simulink model "flightController"  (R2015a)
settings: Solver=ode45  StartTime=0.0  StopTime=10.0  RelTol=1e-3
InitFcn:
  | initSimulation
values from neighbouring files (symbols this model uses):
  maxPitch = 20    [initSimulation.m]
undefined symbols (not defined in the file or in its folder): drawAircraft, forces_moments, P, plotmavstatevariables
libraries: simulink_extras x2
settings Model: Creator=Ludger Heide  LastModifiedBy=Ludger Heide

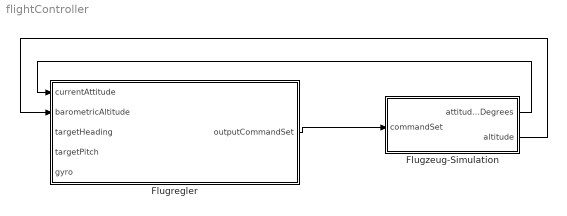
== system flightController ==
  Flugregler : Subsystem  TreatAsAtomicUnit=on
  Flugzeug-Simulation : Subsystem
  wires:
  Flugregler/1(outputCommandSet) -> Flugzeug-Simulation/1(commandSet)
  Flugzeug-Simulation/1(attitudeDegrees) -> Flugregler/1(currentAttitude)
  Flugzeug-Simulation/2(altitude) -> Flugregler/2(barometricAltitude)

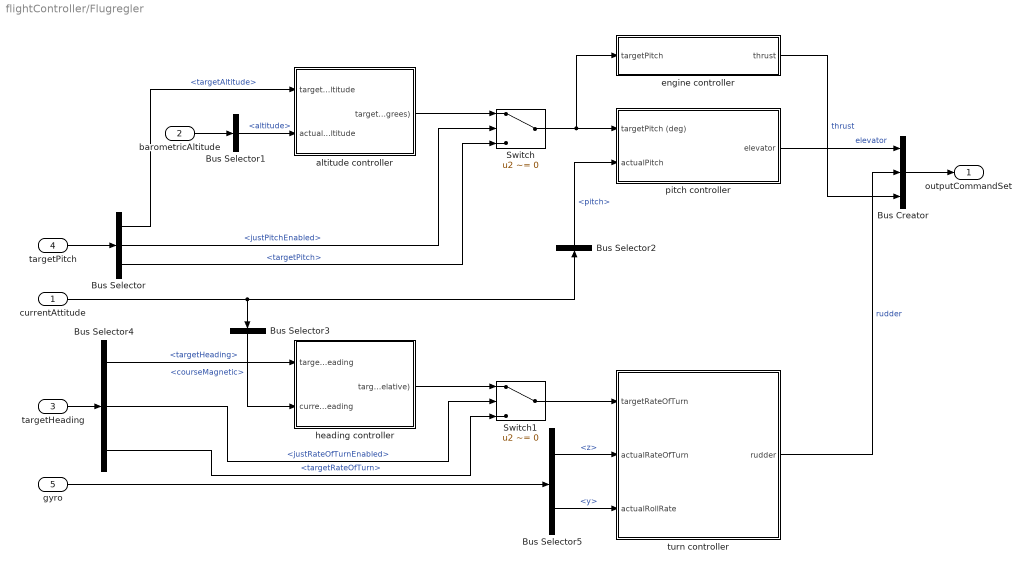
== system flightController/Flugregler ==
  currentAttitude : Inport  OutDataTypeStr=Bus: currentAttitude
  barometricAltitude : Inport  Port=2  OutDataTypeStr=Bus: barometricAltitude
  targetHeading : Inport  Port=3  OutDataTypeStr=Bus: targetHeading
  targetPitch : Inport  Port=4  OutDataTypeStr=Bus: targetPitch
  gyro : Inport  Port=5  OutDataTypeStr=Bus: currentGyro
  Bus Creator : BusCreator  Inputs='elevator','rudder','thrust'  OutDataTypeStr=Bus: outputCommandSet
  Bus Selector : BusSelector  OutputSignals=targetAltitude,justPitchEnabled,targetPitch
  Bus Selector1 : BusSelector  OutputSignals=altitude
  Bus Selector2 : BusSelector  OutputSignals=pitch
  Bus Selector3 : BusSelector  OutputSignals=courseMagnetic
  Bus Selector4 : BusSelector  OutputSignals=targetHeading,justRateOfTurnEnabled,targetRateOfTurn
  Bus Selector5 : BusSelector  OutputSignals=z,y
  Switch : Switch  Criteria=u2 ~= 0
  Switch1 : Switch  Criteria=u2 ~= 0
  altitude controller : Subsystem
  engine controller : Subsystem
  heading controller : Subsystem
  pitch controller : Subsystem
  turn controller : Subsystem
  outputCommandSet : Outport  OutDataTypeStr=Bus: outputCommandSet
  wires:
  Switch/1 -> engine controller/1(targetPitch), pitch controller/1(targetPitch (deg))
  altitude controller/1(targetPitch (degrees)) -> Switch/1
  targetPitch/1 -> Bus Selector/1
  Bus Selector/2 -> Switch/2  "<justPitchEnabled>"
  Bus Selector/3 -> Switch/3  "<targetPitch>"
  Bus Selector/1 -> altitude controller/1(targetAltitude)  "<targetAltitude>"
  barometricAltitude/1 -> Bus Selector1/1
  Bus Selector1/1 -> altitude controller/2(actualAltitude)  "<altitude>"
  Bus Selector2/1 -> pitch controller/2(actualPitch)  "<pitch>"
  currentAttitude/1 -> Bus Selector3/1, Bus Selector2/1
  engine controller/1(thrust) -> Bus Creator/3  "thrust"
  pitch controller/1(elevator) -> Bus Creator/1  "elevator"
  Bus Selector3/1 -> heading controller/2(currentHeading)  "<courseMagnetic>"
  targetHeading/1 -> Bus Selector4/1
  Bus Selector4/1 -> heading controller/1(targetHeading)  "<targetHeading>"
  heading controller/1(targetRateOfTurn (relative)) -> Switch1/1
  Switch1/1 -> turn controller/1(targetRateOfTurn)
  Bus Selector4/2 -> Switch1/2  "<justRateOfTurnEnabled>"
  Bus Selector4/3 -> Switch1/3  "<targetRateOfTurn>"
  turn controller/1(rudder) -> Bus Creator/2  "rudder"
  Bus Creator/1 -> outputCommandSet/1
  Bus Selector5/1 -> turn controller/2(actualRateOfTurn)  "<z>"
  Bus Selector5/2 -> turn controller/3(actualRollRate)  "<y>"
  gyro/1 -> Bus Selector5/1

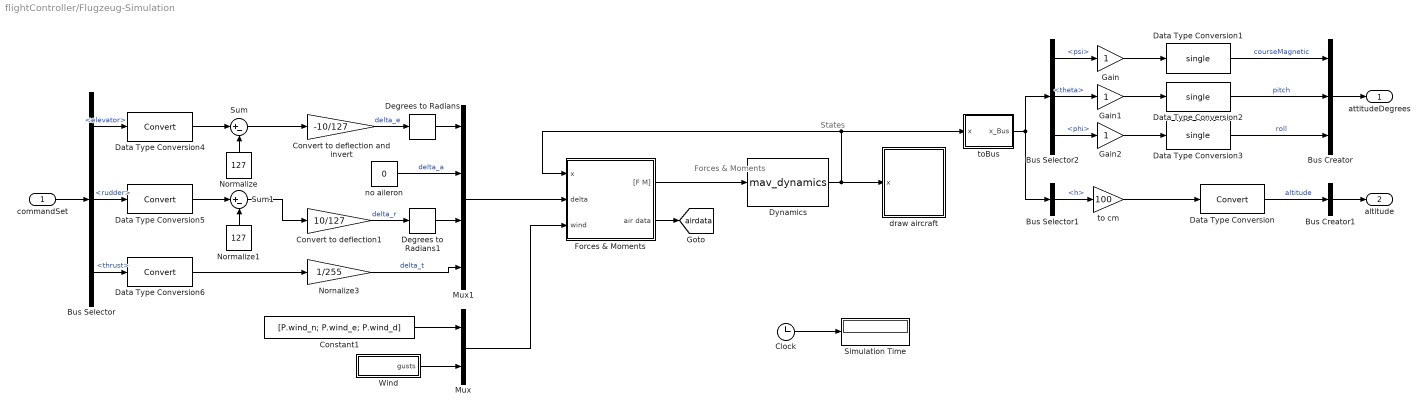
== system flightController/Flugzeug-Simulation ==
  note: Forces & Moments
  note: States
  commandSet : Inport  OutDataTypeStr=Bus: outputCommandSet
  Bus Creator : BusCreator  Inputs='courseMagnetic','pitch','roll'  OutDataTypeStr=Bus: currentAttitude
  Bus Creator1 : BusCreator  Inputs='altitude'  OutDataTypeStr=Bus: barometricAltitude
  Bus Selector : BusSelector  OutputSignals=elevator,rudder,thrust
  Bus Selector1 : BusSelector  OutputSignals=h
  Bus Selector2 : BusSelector  OutputSignals=psi,theta,phi
  Clock : Clock
  Constant1 : Constant  Value=[P.wind_n; P.wind_e; P.wind_d]
  Convert to deflection and invert : Gain  Gain=-10/127
  Convert to deflection1 : Gain  Gain=10/127
  Data Type Conversion{,4..6} (4 alike) : DataTypeConversion
  Data Type Conversion1 : DataTypeConversion  OutDataTypeStr=single
  Data Type Conversion2 : DataTypeConversion  OutDataTypeStr=single
  Data Type Conversion3 : DataTypeConversion  OutDataTypeStr=single
  Degrees to Radians : simulink_extras/Transformations/Degrees to Radians
  Degrees to Radians1 : simulink_extras/Transformations/Degrees to Radians
  Dynamics : S-Function  FunctionName=mav_dynamics  Parameters=P
  Forces & Moments : Subsystem
  Gain : Gain
  Gain1 : Gain
  Gain2 : Gain
  Mux : Mux  Inputs=2
  Mux1 : Mux
  Normalize : Constant  Value=127
  Normalize1 : Constant  Value=127
  Nornalize3 : Gain  Gain=1/255
  Simulation Time : Display
  Sum : Sum  Inputs=|+-
  Sum1 : Sum  Inputs=|+-
  Wind : Subsystem
  draw aircraft : Subsystem
      mask Display: image(imread('tv.jpg'))
  no aileron : Constant  Value=0
  to cm : Gain  Gain=100
  toBus : Subsystem
  attitudeDegrees : Outport  OutDataTypeStr=Bus: currentAttitude
  altitude : Outport  Port=2  OutDataTypeStr=Bus: barometricAltitude
  tag scope: airdata=global
  wires:
  Dynamics/1 -> draw aircraft/1(x), toBus/1(x), Forces & Moments/1(x)
  Convert to deflection1/1 -> Degrees to Radians1/1  "delta_r"
  Convert to deflection and invert/1 -> Degrees to Radians/1  "delta_e"
  Mux1/1 -> Forces & Moments/2(delta)
  Forces & Moments/1("[F M]") -> Dynamics/1
  Clock/1 -> Simulation Time/1
  Mux/1 -> Forces & Moments/3(wind)
  Wind/1(gusts) -> Mux/2
  Constant1/1 -> Mux/1
  Forces & Moments/2(air data) -> [airdata]
  Degrees to Radians/1 -> Mux1/1
  no aileron/1 -> Mux1/2  "delta_a"
  Degrees to Radians1/1 -> Mux1/3
  commandSet/1 -> Bus Selector/1
  Nornalize3/1 -> Mux1/4  "delta_t"
  Bus Selector/1 -> Data Type Conversion4/1  "<elevator>"
  Sum/1 -> Convert to deflection and invert/1
  Normalize/1 -> Sum/2
  Bus Selector/2 -> Data Type Conversion5/1  "<rudder>"
  Sum1/1 -> Convert to deflection1/1
  Normalize1/1 -> Sum1/2
  Bus Selector/3 -> Data Type Conversion6/1  "<thrust>"
  toBus/1(x_Bus) -> Bus Selector2/1, Bus Selector1/1
  Bus Selector2/2 -> Gain1/1  "<theta>"
  Bus Selector2/1 -> Gain/1  "<psi>"
  Bus Selector2/3 -> Gain2/1  "<phi>"
  Gain1/1 -> Data Type Conversion2/1
  Gain2/1 -> Data Type Conversion3/1
  Gain/1 -> Data Type Conversion1/1
  Bus Creator/1 -> attitudeDegrees/1
  to cm/1 -> Data Type Conversion/1
  Bus Selector1/1 -> to cm/1  "<h>"
  Data Type Conversion/1 -> Bus Creator1/1  "altitude"
  Bus Creator1/1 -> altitude/1
  Data Type Conversion1/1 -> Bus Creator/1  "courseMagnetic"
  Data Type Conversion2/1 -> Bus Creator/2  "pitch"
  Data Type Conversion3/1 -> Bus Creator/3  "roll"
  Data Type Conversion4/1 -> Sum/1
  Data Type Conversion5/1 -> Sum1/1
  Data Type Conversion6/1 -> Nornalize3/1

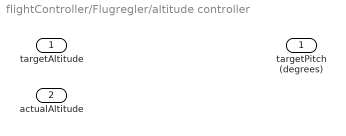
== system flightController/Flugregler/altitude controller ==
  targetAltitude : Inport  OutDataTypeStr=int32
  actualAltitude : Inport  Port=2  OutDataTypeStr=int32
  targetPitch (degrees) : Outport  OutDataTypeStr=int8

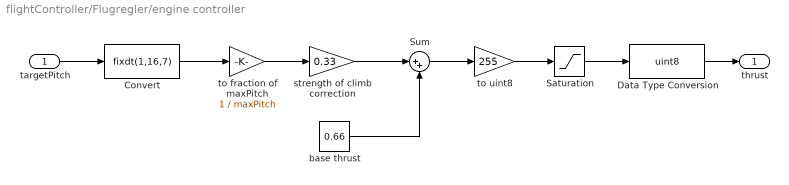
== system flightController/Flugregler/engine controller ==
  targetPitch : Inport  OutDataTypeStr=int8
  Convert : DataTypeConversion  OutMin=-127  OutMax=255  OutDataTypeStr=fixdt(1,16,7)
  Data Type Conversion : DataTypeConversion  OutDataTypeStr=uint8
  Saturation : Saturate  UpperLimit=255  LowerLimit=0
  Sum : Sum  Inputs=|++
  base thrust : Constant  Value=0.66
  strength of climb correction : Gain  Gain=0.33
  to fraction of maxPitch : Gain  Gain=1 / maxPitch
  to uint8 : Gain  Gain=255
  thrust : Outport  OutDataTypeStr=uint8
  wires:
  targetPitch/1 -> Convert/1
  Convert/1 -> to fraction of maxPitch/1
  to fraction of maxPitch/1 -> strength of climb correction/1
  base thrust/1 -> Sum/2
  strength of climb correction/1 -> Sum/1
  Sum/1 -> to uint8/1
  to uint8/1 -> Saturation/1
  Saturation/1 -> Data Type Conversion/1
  Data Type Conversion/1 -> thrust/1

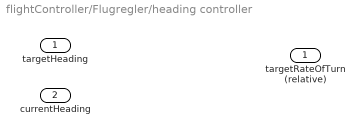
== system flightController/Flugregler/heading controller ==
  targetHeading : Inport  OutDataTypeStr=uint16
  currentHeading : Inport  Port=2  OutDataTypeStr=single
  targetRateOfTurn (relative) : Outport  OutDataTypeStr=int8

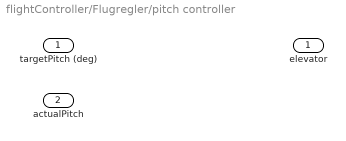
== system flightController/Flugregler/pitch controller ==
  targetPitch (deg) : Inport  OutDataTypeStr=int8
  actualPitch : Inport  Port=2  OutDataTypeStr=single
  elevator : Outport  OutDataTypeStr=uint8

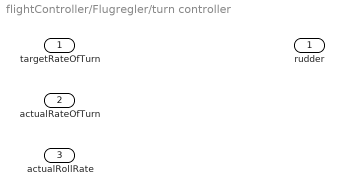
== system flightController/Flugregler/turn controller ==
  targetRateOfTurn : Inport  OutDataTypeStr=int8
  actualRateOfTurn : Inport  Port=2  OutDataTypeStr=single
  actualRollRate : Inport  Port=3  OutDataTypeStr=single
  rudder : Outport  OutDataTypeStr=uint8

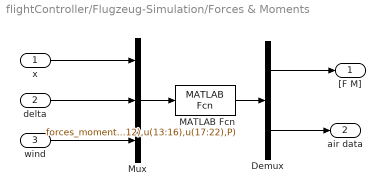
== system flightController/Flugzeug-Simulation/Forces & Moments ==
  x : Inport
  delta : Inport  Port=2
  wind : Inport  Port=3
  Demux : Demux  Outputs=[6;6]
  MATLAB Fcn : MATLABFcn  MATLABFcn=forces_moments(u(1:12),u(13:16),u(17:22),P)  OutputDimensions=12
  Mux : Mux  Inputs=3
  "[F M]" : Outport
  air data : Outport  Port=2
  wires:
  x/1 -> Mux/1
  delta/1 -> Mux/2
  wind/1 -> Mux/3
  MATLAB Fcn/1 -> Demux/1
  Demux/1 -> "[F M]"/1
  Mux/1 -> MATLAB Fcn/1
  Demux/2 -> air data/1

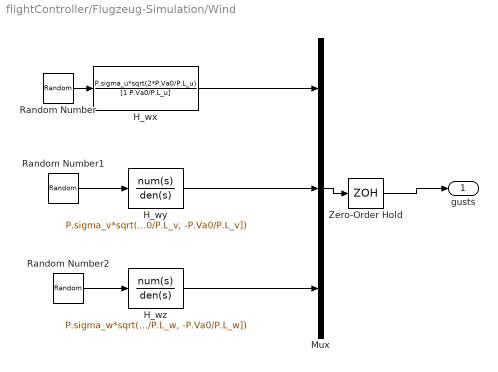
== system flightController/Flugzeug-Simulation/Wind ==
  H_wx : TransferFcn  Numerator=P.sigma_u*sqrt(2*P.Va0/P.L_u)  Denominator=[1 P.Va0/P.L_u]
  H_wy : TransferFcn  Numerator=P.sigma_v*sqrt(3*P.Va0/P.L_v)*[0, 1, P.Va0/sqrt(3)/P.L_v]  Denominator=poly([-P.Va0/P.L_v, -P.Va0/P.L_v])
  H_wz : TransferFcn  Numerator=P.sigma_w*sqrt(3*P.Va0/P.L_w)*[0, 1, P.Va0/sqrt(3)/P.L_w]  Denominator=poly([-P.Va0/P.L_w, -P.Va0/P.L_w])
  Mux : Mux  Inputs=3
  Random Number : RandomNumber  SampleTime=0
  Random Number1 : RandomNumber  SampleTime=0
  Random Number2 : RandomNumber  SampleTime=0
  Zero-Order Hold : ZeroOrderHold  SampleTime=P.Ts
  gusts : Outport
  wires:
  H_wx/1 -> Mux/1
  Random Number/1 -> H_wx/1
  H_wy/1 -> Mux/2
  Random Number1/1 -> H_wy/1
  H_wz/1 -> Mux/3
  Random Number2/1 -> H_wz/1
  Mux/1 -> Zero-Order Hold/1
  Zero-Order Hold/1 -> gusts/1

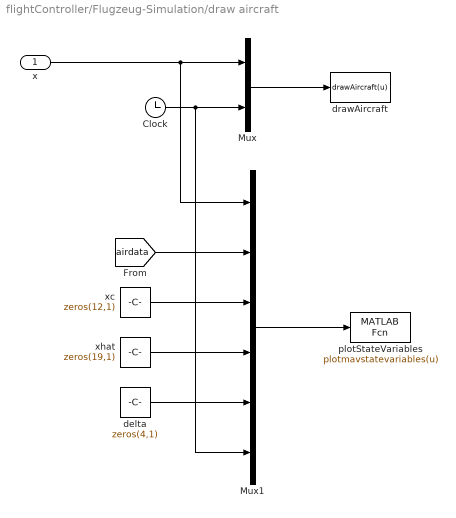
== system flightController/Flugzeug-Simulation/draw aircraft ==
  x : Inport
  Clock : Clock
  Mux : Mux  Inputs=2
  Mux1 : Mux  Inputs=6
  delta : Constant  Value=zeros(4,1)
  drawAircraft : MATLABFcn  MATLABFcn=drawAircraft(u)  OutputDimensions=0  SampleTime=0.1
  plotStateVariables : MATLABFcn  MATLABFcn=plotmavstatevariables(u)  OutputDimensions=0  SampleTime=0.1
  xc : Constant  Value=zeros(12,1)
  xhat : Constant  Value=zeros(19,1)
  wires:
  [airdata] -> Mux1/2
  delta/1 -> Mux1/5
  xc/1 -> Mux1/3
  xhat/1 -> Mux1/4
  Mux1/1 -> plotStateVariables/1
  Clock/1 -> Mux1/6, Mux/2
  x/1 -> Mux1/1, Mux/1
  Mux/1 -> drawAircraft/1

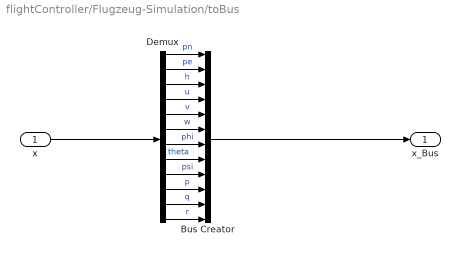
== system flightController/Flugzeug-Simulation/toBus ==
  x : Inport
  Bus Creator : BusCreator  Inputs=12
  Demux : Demux  Outputs=12
  x_Bus : Outport
  wires:
  Demux/7 -> Bus Creator/7  "phi"
  Demux/11 -> Bus Creator/11  "q"
  Demux/10 -> Bus Creator/10  "p"
  Demux/1 -> Bus Creator/1  "pn"
  Demux/5 -> Bus Creator/5  "v"
  Demux/2 -> Bus Creator/2  "pe"
  Demux/4 -> Bus Creator/4  "u"
  Demux/6 -> Bus Creator/6  "w"
  Demux/9 -> Bus Creator/9  "psi"
  Demux/8 -> Bus Creator/8  "theta"
  Demux/12 -> Bus Creator/12  "r"
  Demux/3 -> Bus Creator/3  "h"
  Bus Creator/1 -> x_Bus/1
  x/1 -> Demux/1
